simulink model "naoLinear_junta1"  (R2020a)
settings: Solver=VariableStepAuto  StartTime=0.0  StopTime=9  MaxStep=0.0050  RelTol=1e-3
values from neighbouring files (symbols this model uses):
  K = zinf/deltaVm    [identificacao_junta_1.m]
  Kl = w1/Vm1    (= 40)    [identificacao_junta_1.m]
  phi = K*Vm1-w1    [identificacao_junta_1.m]
  T = 0.01    [identificacao_junta_1.m]
settings Model: Creator=ViniciusSimoes  LastModifiedBy=ViniciusSimoes

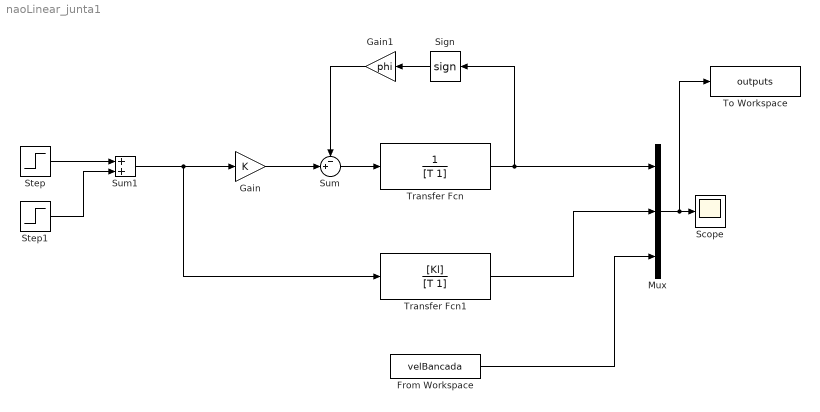
== system naoLinear_junta1 ==
  From Workspace : FromWorkspace  VariableName=velBancada
  Gain : Gain  Gain=K
  Gain1 : Gain  Gain=phi
  Mux : Mux  Inputs=3
  Scope : Scope
  Sign : Signum
  Step : Step  Time=3  After=5  SampleTime=0
  Step1 : Step  Time=6  After=4  SampleTime=0
  Sum : Sum  Inputs=-+|
  Sum1 : Sum
  To Workspace : ToWorkspace  VariableName=outputs  SaveFormat=Timeseries  SampleTime=-1
  Transfer Fcn : TransferFcn  Denominator=[T 1]
  Transfer Fcn1 : TransferFcn  Numerator=[Kl]  Denominator=[T 1]
  wires:
  Gain/1 -> Sum/2
  Sum/1 -> Transfer Fcn/1
  Transfer Fcn/1 -> Mux/1, Sign/1
  Sign/1 -> Gain1/1
  Gain1/1 -> Sum/1
  Sum1/1 -> Transfer Fcn1/1, Gain/1
  Step/1 -> Sum1/1
  Step1/1 -> Sum1/2
  Transfer Fcn1/1 -> Mux/2
  Mux/1 -> To Workspace/1, Scope/1
  From Workspace/1 -> Mux/3
